simulink library "MOT_lib"  (R2015a)
settings: Solver=ode45  StartTime=0.0  StopTime=10.0  RelTol=1e-3
values from neighbouring files (symbols this model uses):
  MOT = MOTmod    [setup_mot.m]
settings Model: Creator=Andrew  LastModifiedBy=Andrew

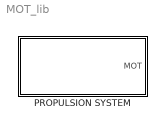
== system MOT_lib ==
  PROPULSION SYSTEM : Subsystem

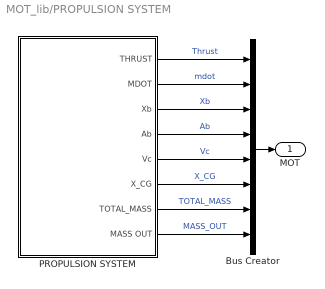
== system MOT_lib/PROPULSION SYSTEM ==
  Bus Creator : BusCreator  Inputs=8
  PROPULSION SYSTEM : Subsystem
  MOT : Outport
  wires:
  PROPULSION SYSTEM/1(THRUST) -> Bus Creator/1  "Thrust"
  PROPULSION SYSTEM/2(MDOT) -> Bus Creator/2  "mdot"
  Bus Creator/1 -> MOT/1
  PROPULSION SYSTEM/4(Ab) -> Bus Creator/4  "Ab"
  PROPULSION SYSTEM/8(MASS OUT) -> Bus Creator/8  "MASS_OUT"
  PROPULSION SYSTEM/3(Xb) -> Bus Creator/3  "Xb"
  PROPULSION SYSTEM/5(Vc) -> Bus Creator/5  "Vc"
  PROPULSION SYSTEM/6(X_CG) -> Bus Creator/6  "X_CG"
  PROPULSION SYSTEM/7(TOTAL_MASS) -> Bus Creator/7  "TOTAL_MASS"

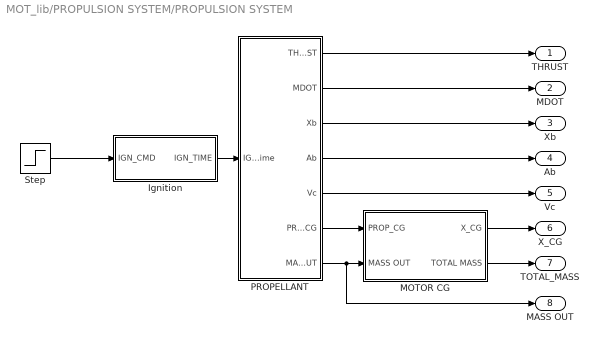
== system MOT_lib/PROPULSION SYSTEM/PROPULSION SYSTEM ==
  Ignition : Subsystem
  MOTOR CG : Subsystem
  PROPELLANT : Subsystem
  Step : Step  Time=0.005  SampleTime=0
  THRUST : Outport
  MDOT : Outport  Port=2
  Xb : Outport  Port=3
  Ab : Outport  Port=4
  Vc : Outport  Port=5
  X_CG : Outport  Port=6
  TOTAL_MASS : Outport  Port=7
  MASS OUT : Outport  Port=8
  wires:
  PROPELLANT/1(THRUST) -> THRUST/1
  PROPELLANT/2(MDOT) -> MDOT/1
  PROPELLANT/7(MASS OUT) -> MASS OUT/1, MOTOR CG/2(MASS OUT)
  PROPELLANT/3(Xb) -> Xb/1
  PROPELLANT/4(Ab) -> Ab/1
  PROPELLANT/5(Vc) -> Vc/1
  Ignition/1(IGN_TIME) -> PROPELLANT/1(IGN_Time)
  PROPELLANT/6("PROP_CG ") -> MOTOR CG/1(PROP_CG)
  MOTOR CG/1(X_CG) -> X_CG/1
  MOTOR CG/2(TOTAL MASS) -> TOTAL_MASS/1
  Step/1 -> Ignition/1(IGN_CMD)

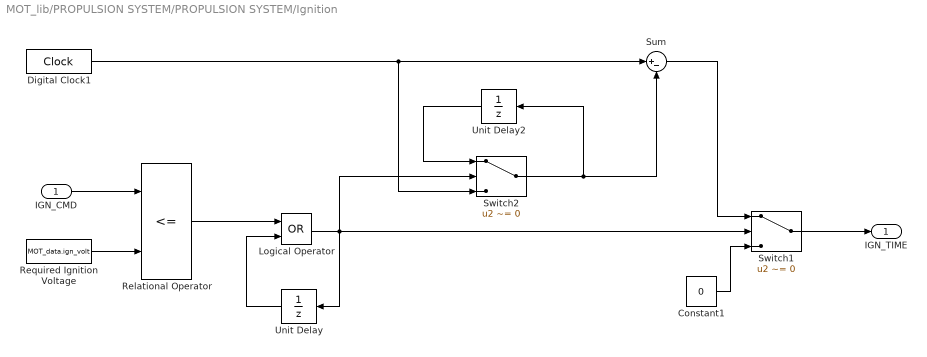
== system MOT_lib/PROPULSION SYSTEM/PROPULSION SYSTEM/Ignition ==
  IGN_CMD : Inport
  Constant1 : Constant  Value=0
  Digital Clock1 : DigitalClock  SampleTime=0.0025
  Logical Operator : Logic  Operator=OR  AllPortsSameDT=off  OutDataTypeStr=boolean
  Relational Operator : RelationalOperator  Operator=<=  OutDataTypeStr=boolean
  Required Ignition Voltage : FromWorkspace  VariableName=MOT_data.ign_volt  SampleTime=0
  Sum : Sum  Inputs=|+-
  Switch1 : Switch  Criteria=u2 ~= 0
  Switch2 : Switch  Criteria=u2 ~= 0
  Unit Delay : UnitDelay  SampleTime=-1
  Unit Delay2 : UnitDelay  SampleTime=-1
  IGN_TIME : Outport
  wires:
  IGN_CMD/1 -> Relational Operator/1
  Required Ignition Voltage/1 -> Relational Operator/2
  Relational Operator/1 -> Logical Operator/1
  Unit Delay/1 -> Logical Operator/2
  Constant1/1 -> Switch1/3
  Logical Operator/1 -> Switch1/2, Unit Delay/1, Switch2/2
  Digital Clock1/1 -> Switch2/3, Sum/1
  Sum/1 -> Switch1/1
  Switch1/1 -> IGN_TIME/1
  Switch2/1 -> Unit Delay2/1, Sum/2
  Unit Delay2/1 -> Switch2/1

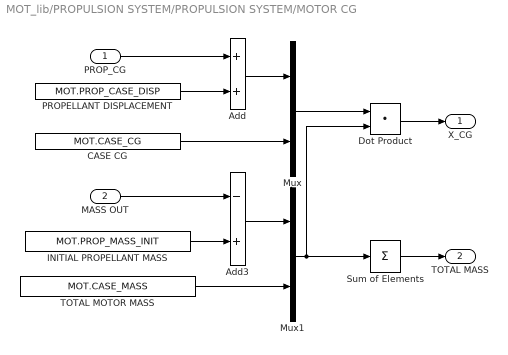
== system MOT_lib/PROPULSION SYSTEM/PROPULSION SYSTEM/MOTOR CG ==
  PROP_CG : Inport
  MASS OUT : Inport  Port=2
  Add : Sum
  Add3 : Sum  Inputs=-+
  CASE CG : Constant  Value=MOT.CASE_CG
  Dot Product : DotProduct  InputSameDT=on  OutDataTypeStr=Inherit: Inherit via internal rule
  INITIAL PROPELLANT MASS : Constant  Value=MOT.PROP_MASS_INIT
  Mux : Mux  Inputs=2
  Mux1 : Mux  Inputs=2
  PROPELLANT DISPLACEMENT : Constant  Value=MOT.PROP_CASE_DISP
  Sum of Elements : Sum  Inputs=+
  TOTAL MOTOR MASS : Constant  Value=MOT.CASE_MASS
  X_CG : Outport
  TOTAL MASS : Outport  Port=2
  wires:
  PROP_CG/1 -> Add/1
  PROPELLANT DISPLACEMENT/1 -> Add/2
  Add/1 -> Mux/1
  CASE CG/1 -> Mux/2
  Dot Product/1 -> X_CG/1
  Mux/1 -> Dot Product/1
  Mux1/1 -> Dot Product/2, Sum of Elements/1
  TOTAL MOTOR MASS/1 -> Mux1/2
  Add3/1 -> Mux1/1
  MASS OUT/1 -> Add3/1
  INITIAL PROPELLANT MASS/1 -> Add3/2
  Sum of Elements/1 -> TOTAL MASS/1

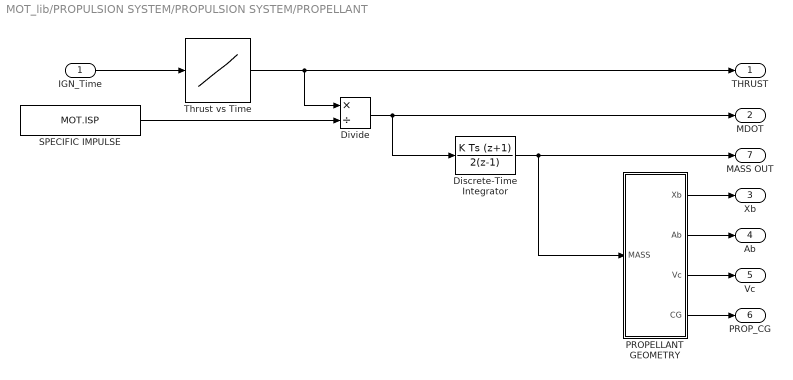
== system MOT_lib/PROPULSION SYSTEM/PROPULSION SYSTEM/PROPELLANT ==
  IGN_Time : Inport
  Discrete-Time Integrator : DiscreteIntegrator  IntegratorMethod=Integration: Trapezoidal  InitialConditionSetting=State (most efficient)  SampleTime=-1
  Divide : Product  Inputs=*/
  PROPELLANT GEOMETRY : Subsystem
  SPECIFIC IMPULSE : Constant  Value=MOT.ISP
  Thrust vs Time : Lookup_n-D  NumberOfTableDimensions=1  BreakpointsForDimension1=MOT.THRUST_TABLE_X  Table=MOT.THRUST_TABLE_Y  InternalRulePriority=Speed  RndMeth=Simplest  InputSameDT=on
  THRUST : Outport
  MDOT : Outport  Port=2
  Xb : Outport  Port=3
  Ab : Outport  Port=4
  Vc : Outport  Port=5
  "PROP_CG " : Outport  Port=6
  MASS OUT : Outport  Port=7
  wires:
  PROPELLANT GEOMETRY/2(Ab) -> Ab/1
  Discrete-Time Integrator/1 -> PROPELLANT GEOMETRY/1(MASS), MASS OUT/1
  PROPELLANT GEOMETRY/3(Vc) -> Vc/1
  PROPELLANT GEOMETRY/4(CG) -> "PROP_CG "/1
  PROPELLANT GEOMETRY/1(Xb) -> Xb/1
  IGN_Time/1 -> Thrust vs Time/1
  Thrust vs Time/1 -> THRUST/1, Divide/1
  SPECIFIC IMPULSE/1 -> Divide/2
  Divide/1 -> MDOT/1, Discrete-Time Integrator/1

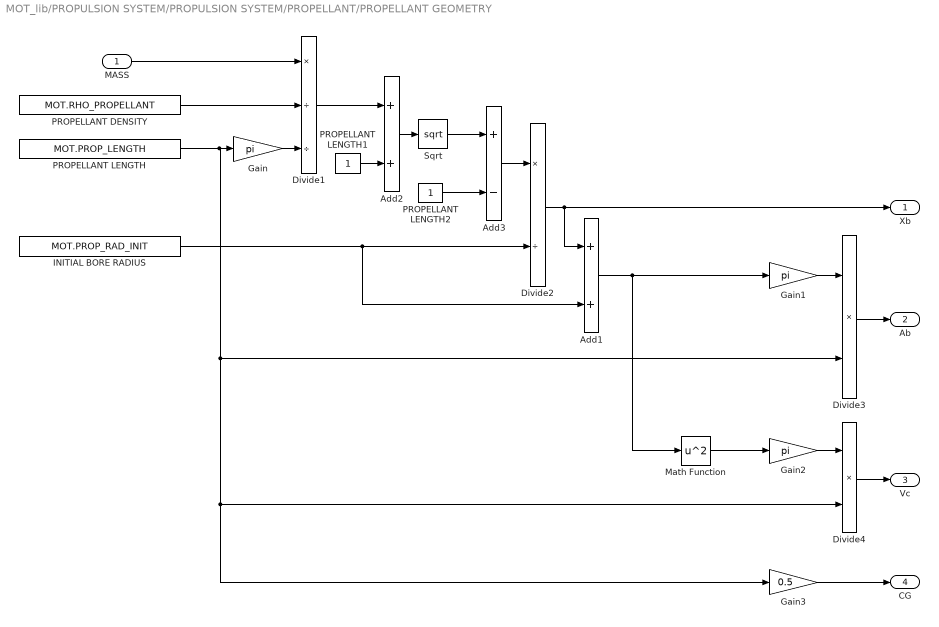
== system MOT_lib/PROPULSION SYSTEM/PROPULSION SYSTEM/PROPELLANT/PROPELLANT GEOMETRY ==
  MASS : Inport
  Add1 : Sum
  Add2 : Sum
  Add3 : Sum  Inputs=+-
  Divide1 : Product  Inputs=*//
  Divide2 : Product  Inputs=*/
  Divide3 : Product  Inputs=**
  Divide4 : Product  Inputs=**
  Gain : Gain  Gain=pi
  Gain1 : Gain  Gain=pi
  Gain2 : Gain  Gain=pi
  Gain3 : Gain  Gain=0.5
  INITIAL BORE RADIUS : Constant  Value=MOT.PROP_RAD_INIT
  Math Function : Math  Operator=square  SaturateOnIntegerOverflow=on
  PROPELLANT DENSITY : Constant  Value=MOT.RHO_PROPELLANT
  PROPELLANT LENGTH : Constant  Value=MOT.PROP_LENGTH
  PROPELLANT LENGTH1 : Constant
  PROPELLANT LENGTH2 : Constant
  Sqrt : Sqrt  SaturateOnIntegerOverflow=on
  Xb : Outport
  Ab : Outport  Port=2
  Vc : Outport  Port=3
  CG : Outport  Port=4
  wires:
  PROPELLANT DENSITY/1 -> Divide1/2
  Gain/1 -> Divide1/3
  Divide1/1 -> Add2/1
  Add2/1 -> Sqrt/1
  Sqrt/1 -> Add3/1
  PROPELLANT LENGTH2/1 -> Add3/2
  PROPELLANT LENGTH1/1 -> Add2/2
  PROPELLANT LENGTH/1 -> Divide3/2, Gain3/1, Divide4/2, Gain/1
  MASS/1 -> Divide1/1
  Add3/1 -> Divide2/1
  Divide2/1 -> Xb/1, Add1/1
  INITIAL BORE RADIUS/1 -> Add1/2, Divide2/2
  Add1/1 -> Gain1/1, Math Function/1
  Gain1/1 -> Divide3/1
  Divide3/1 -> Ab/1
  Divide4/1 -> Vc/1
  Gain2/1 -> Divide4/1
  Math Function/1 -> Gain2/1
  Gain3/1 -> CG/1
